simulink model "ahlb_ut"  (R2013b)
settings: Solver=FixedStepDiscrete  StartTime=0.0  StopTime=inf  FixedStep=0.005  RelTol=1e-3
libraries: siltestlib x4, ahlb x1, simulink x1
settings Model: Creator=12103  LastModifiedBy=12103

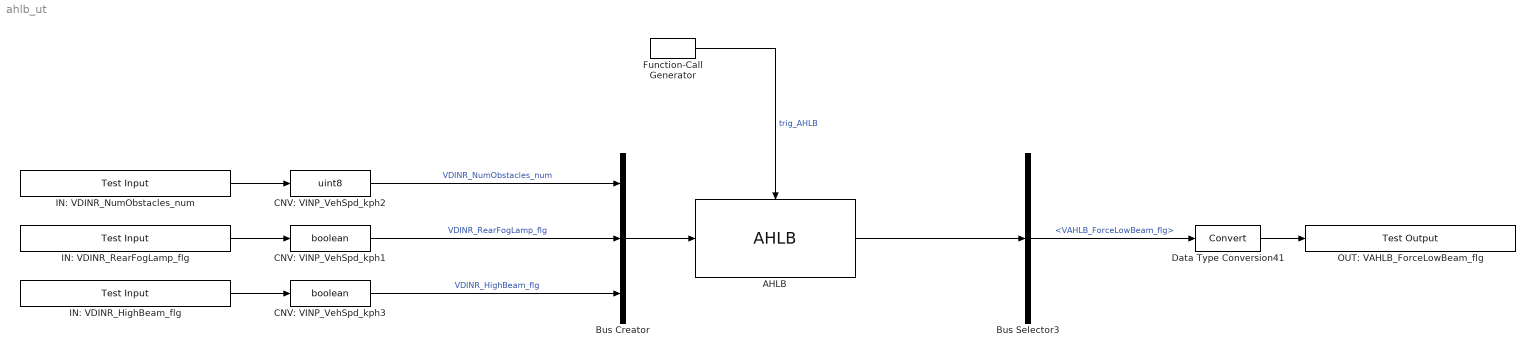
== system ahlb_ut ==
  AHLB : ahlb/AHLB
  Bus Creator : BusCreator  Inputs=3
  Bus Selector3 : BusSelector  OutputSignals=VAHLB_ForceLowBeam_flg
  CNV: VINP_VehSpd_kph1 : DataTypeConversion  OutDataTypeStr=boolean
  CNV: VINP_VehSpd_kph2 : DataTypeConversion  OutDataTypeStr=uint8
  CNV: VINP_VehSpd_kph3 : DataTypeConversion  OutDataTypeStr=boolean
  Data Type Conversion41 : DataTypeConversion
  Function-Call Generator : simulink/Ports & Subsystems/Function-Call Generator  sample_time=5E-3  numberOfIterations=1
  IN: VDINR_HighBeam_flg : siltestlib/Test Input  varname=VDINR_HighBeam_flg  sampletime=-1
  IN: VDINR_NumObstacles_num : siltestlib/Test Input  varname=VDINR_NumObstacles_num  sampletime=-1
  IN: VDINR_RearFogLamp_flg : siltestlib/Test Input  varname=VDINR_RearFogLamp_flg  sampletime=-1
  OUT: VAHLB_ForceLowBeam_flg : siltestlib/Test Output  varname=VAHLB_ForceLowBeam_flg  sampletime=-1
  wires:
  Data Type Conversion41/1 -> OUT: VAHLB_ForceLowBeam_flg/1
  Bus Selector3/1 -> Data Type Conversion41/1  "<VAHLB_ForceLowBeam_flg>"
  Function-Call Generator/1 -> AHLB/Trigger  "trig_AHLB"
  AHLB/1 -> Bus Selector3/1
  IN: VDINR_HighBeam_flg/1 -> CNV: VINP_VehSpd_kph3/1
  IN: VDINR_RearFogLamp_flg/1 -> CNV: VINP_VehSpd_kph1/1
  IN: VDINR_NumObstacles_num/1 -> CNV: VINP_VehSpd_kph2/1
  CNV: VINP_VehSpd_kph2/1 -> Bus Creator/1  "VDINR_NumObstacles_num"
  CNV: VINP_VehSpd_kph1/1 -> Bus Creator/2  "VDINR_RearFogLamp_flg"
  CNV: VINP_VehSpd_kph3/1 -> Bus Creator/3  "VDINR_HighBeam_flg"
  Bus Creator/1 -> AHLB/1
